simulink model "time_delay_discrete_model"  (R2023b)
settings: Solver=VariableStepAuto  StartTime=0.0  StopTime=20  RelTol=1e-3
values from neighbouring files (symbols this model uses):
  A = [Aaa Aab; Aba Abb]    [compensated_minimum_order_controller.m]    (also in compensated_observer_controller.m = [A Bv*Cc; zeros(1, 3) Ac]; direct_comp_calib.m; direct_compensated_minimum_order_controller.m; experiment_calc.m)
  Ad = Md(1:3, 1:3)    [experiment_calc.m]    (also in experiment_sym.m; scalar_lambert_W.m = -[0 0; -kc/km*wn^2 0]; simple_time_delay_discrete.m = Md(1:2, 1:2); simple_time_delay_sym.m = Md(1:2, 1:2))
  Aimp = [0 1; -Ke/Me -Be/Me]    [experiment_calc.m]    (also in experiment_sym.m; time_delay_continuous.m; time_delay_continuous_sym.m; time_delay_discrete.m)
  B = -8*P.*M*0.05    [comp_controller_param_map.m]    (also in compensated_minimum_order_controller.m = [Bt Bv]; compensated_observer_controller.m = [0 0; 1/J 0; 0 1/L]; direct_comp_calib.m = [Bt Bv]; direct_compensated_minimum_order_controller.m = [Bt Bv])
  Bd = Md(1:3, 4:end)    [experiment_calc.m]    (also in experiment_sym.m; simple_time_delay_discrete.m = Md(1:2, 3:end); simple_time_delay_sym.m = Md(1:2, 3:end); time_delay_discrete.m = Atilde\(Ad-eye(2))*Btilde)
  Bimp = [0 0; Ke/Me 1/Me]    [experiment_calc.m]    (also in experiment_sym.m; time_delay_continuous.m; time_delay_continuous_sym.m; time_delay_discrete.m)
  C = [1 0 0]    [compensated_minimum_order_controller.m]    (also in compensated_observer_controller.m = [C 0]; direct_comp_calib.m; direct_compensated_minimum_order_controller.m; experiment_calc.m)
  Cd = C    [experiment_calc.m]    (also in experiment_sym.m; simple_time_delay_discrete.m; simple_time_delay_sym.m; time_delay_discrete.m = Ctilde)
  Cimp = [1 0]    [experiment_calc.m]    (also in experiment_sym.m = eye(2); time_delay_continuous.m = eye(2); time_delay_continuous_sym.m; time_delay_discrete.m = eye(2))
  D = [0 0]    [compensated_minimum_order_controller.m]    (also in compensated_observer_controller.m = 0; direct_comp_calib.m; direct_compensated_minimum_order_controller.m; experiment_calc.m)
  Dd = D    [experiment_calc.m]    (also in experiment_sym.m; simple_time_delay_discrete.m = 0; simple_time_delay_sym.m = 0; time_delay_discrete.m = Dtilde)
  Dimp = zeros(2)    [experiment_calc.m]    (also in experiment_sym.m; time_delay_continuous.m; time_delay_continuous_sym.m; time_delay_discrete.m)
  nutildei = nui - ei    [experiment_sym.m]    (also in simple_time_delay_discrete.m; time_delay_continuous.m; time_delay_discrete.m)
  t_d = 0.001    [experiment_sym.m]    (also in time_delay_discrete.m = 0.2)
  xi = [1; 0; 0]    [experiment_sym.m]    (also in simple_time_delay_discrete.m = [1; 0]; time_delay_continuous.m = [0; 0; 0]; time_delay_discrete.m = [0; 0; 0]; time_delay_discrete_fourier.m)
settings Model: Creator=tamas  LastModifiedBy=tamas

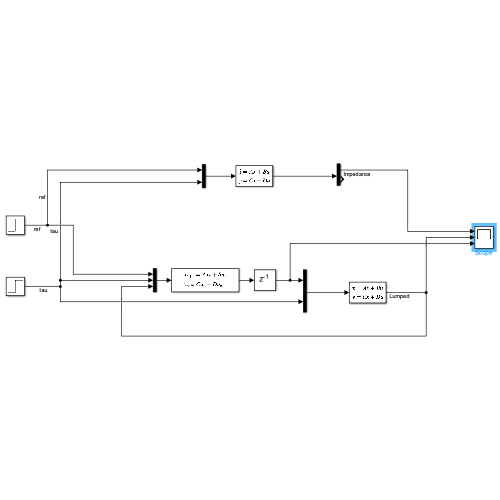
[thumbnail: Simulink's stored preview of the top-level diagram]
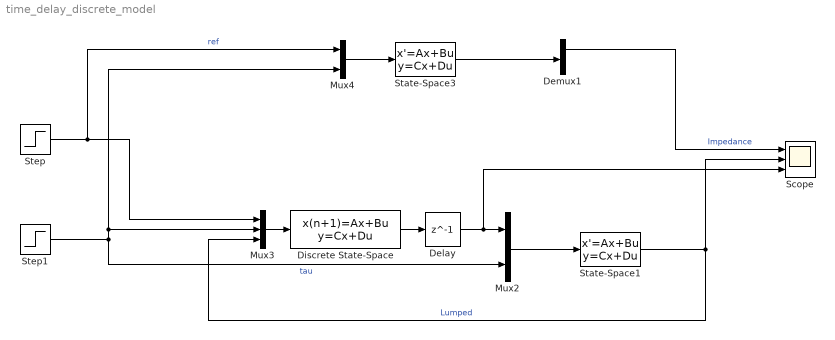
== system time_delay_discrete_model ==
  Delay : Delay  DelayLength=1  InitialCondition=0
  Demux1 : Demux  Outputs=2
  Discrete State-Space : DiscreteStateSpace  A=Ad  B=Bd  C=Cd  D=Dd  InitialCondition=nutildei  SampleTime=t_d
  Mux2 : Mux  Inputs=2
  Mux3 : Mux  Inputs=3
  Mux4 : Mux  Inputs=2
  Scope : Scope  NumInputPorts=3
  State-Space1 : StateSpace  A=A  B=B  C=C  D=D  InitialCondition=xi
  State-Space3 : StateSpace  A=Aimp  B=Bimp  C=Cimp  D=Dimp  InitialCondition=xi(1:2)
  Step : Step  Time=0  SampleTime=0
  Step1 : Step  Time=0  After=0  SampleTime=0
  wires:
  State-Space1/1 -> Scope/2, Mux3/3  "Lumped"
  Mux2/1 -> State-Space1/1
  Mux3/1 -> Discrete State-Space/1
  Mux4/1 -> State-Space3/1
  Step1/1 -> Mux3/2, Mux4/2, Mux2/2  "tau"
  Step/1 -> Mux3/1, Mux4/1  "ref"
  State-Space3/1 -> Demux1/1
  Delay/1 -> Scope/3, Mux2/1
  Discrete State-Space/1 -> Delay/1
  Demux1/1 -> Scope/1  "Impedance"
